simulink model "fir_core"  (Simulink 7.4)
settings: Solver=ode45  StartTime=0.0  StopTime=10.0  RelTol=1e-3
undefined symbols (not defined in the file or in its folder): pfb_coeff_gen_calc
libraries: xbsIndex_r4 x708, casper_library_delays x96
(part 1 of 9)
settings Model: Creator=rprimian  LastModifiedBy=rprimian
settings DebuggingCC: StrictBusMsg=ErrorLevel1

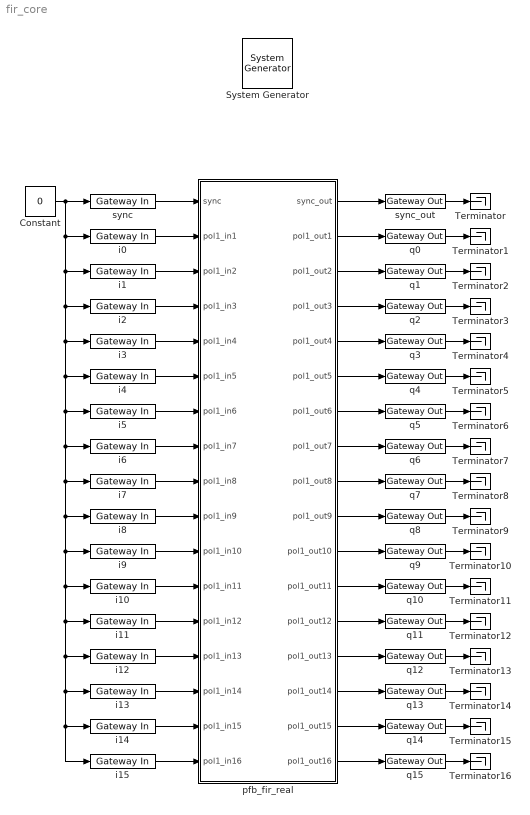
== system fir_core ==
  " System Generator" : xbsIndex_r4/ System Generator  Tag=genX  SystemSampleTime=-1  xilinxfamily=virtex6  part=xc6vsx475t  speed=-1  package=ff1759  synthesis_tool=XST  clock_wrapper=Clock Enables  directory=./fir_core  testbench=off  simulink_period=1  sysclk_period=10  dcm_input_clock_period=100  incr_netlist=off  trim_vbits=Everywhere in SubSystem  dbl_ovrd=According to Block Masks  core_generation=According to Block Masks  run_coregen=off  deprecated_control=off  eval_field=0  block_type=sysgen
      settings: block_version=11.4
  Constant : Constant  Value=0
  Terminator{,1..16} (17 alike) : Terminator
  i{0..15} (16 alike) : xbsIndex_r4/Gateway In  arith_type="Signed  (2's comp)"  n_bits=8  bin_pt=7  quantization="Round  (unbiased: +/- Inf)"  overflow=Saturate  period=1  dbl_ovrd=off  timing_constraint=None  locs_specified=off  LOCs={}  hdl_port=on  block_type=gatewayin
      settings: infoedit="Gateway in block.  Converts inputs of type Simulink integer, double and fixed point to  Xilinx fixed point type.<br><br>Hardware notes:  In hardware these blocks become top level input ports."  block_version=11.4
  pfb_fir_real : Subsystem  AncestorBlock=casper_library_pfbs/pfb_fir_real  mask(pfb_fir_real){PFBSize=15, TotalTaps=4, WindowType=hamming, n_inputs=4, MakeBiplex=off, BitWidthIn=8, BitWidthOut=18, CoeffBitWidth=18, CoeffDistMem=off, add_latency=3, mult_latency=3, bram_latency=3, fan_latency=1, conv_latency=3, quantization=Round  (unbiased: +/- Inf), fwidth=1, mult_spec=2, adder_folding=off, adder_imp=Behavioral, coeffs_share=off}
      mask prompts: PFBSize "Size of PFB: (2^? pnts)"; TotalTaps "Total Number of Taps:"; WindowType "Windowing Function:"; n_inputs "Number of Simultaneous Inputs: (2^?)"; MakeBiplex "Make Biplex?"; BitWidthIn "Input Bitwidth:"; BitWidthOut "Output Bitwidth:"; CoeffBitWidth "Coefficient Bitwidth:"; CoeffDistMem "Use Distributed Memory for Coeffs"; add_latency "Add Latency"; mult_latency "Mult Latency"; bram_latency "BRAM Latency"; fan_latency "Fanout latency"; conv_latency "Convert latency"; quantization "Quantization Behavior"; fwidth "Bin Width Scaling (normal=1)"; mult_spec "Multiplier specification (0=core, 1=embedded, 2=behavioural) (left=1st tap, or just one value)"; adder_folding "Fold adders into DSPs"; adder_imp "Adder implementation"; coeffs_share "Share coefficients between polarisations (use less BRAM)?"
      mask help:
      | Fold adders into DSPs: Causes adders to be absorbed into DSP blocks (supported in Virtex5)
      | Adder implementation: Cores using Fabric or DSP48 or behavioral HDL
      mask init:
      | pfb_fir_real_init(gcb, ...
      |     'PFBSize', PFBSize, ...
      |     'TotalTaps', TotalTaps, ...
      |     'WindowType', WindowType, ...
      |     'n_inputs', n_inputs, ...
      |     'MakeBiplex', MakeBiplex, ...
      |     'BitWidthIn', BitWidthIn, ...
      |     'BitWidthOut', BitWidthOut, ...
      |     'CoeffBitWidth', CoeffBitWidth, ...
      |     'CoeffDistMem', CoeffDistMem, ...
      |     'add_latency', add_latency, ...
      |     'mult_latency', mult_latency, ...
      |     'bram_latency', bram_latency, ...
      |     'fan_latency', fan_latency, ...
      |     'conv_latency', conv_latency, ...
      |     'quantization', quantization, ...
      |     'fwidth', fwidth, ...
      |     'mult_spec', mult_spec, ...
      |     'adder_folding', adder_folding, ...
      |     'adder_imp', adder_imp, ...
      |     'coeffs_share', coeffs_share);
      settings: AttributesFormatString=taps=4, add_latency=3
      mask Help: eval('xlWeb(''http://casper.berkeley.edu/wiki/Pfb_fir_real'')')
      mask StyleString: edit,edit,popup(bartlett|barthannwin|blackman|blackmanharris|bohamwin|chebwin|flattopwin|gausswin|hamming|hann|kaiser|nuttallwin|parzenwin|rectwin|tukeywin|triang|userwindow),edit,checkbox,edit,edit,edit,checkbox,edit,edit,edit,edit,edit,popup(Truncate|Round  (unbiased: +/- Inf)|Round  (unbiased: Even Values)),edit,edit,checkbox,popup(Behavioral|Fabric|DSP48),checkbox
      mask CallbackString:
      | |%num_taps = eval(get_param(gcb, 'TotalTaps'));
      | %old_vec = eval(get_param(gcb, 'mult_spec'));=-0l
      | 
      | %vec = 2.*ones(1,num_taps);
      | %old_size = length(old_vec);
      | 
      | %if(old_size <= num_taps),
      | %    new_size = old_size;
      | %else,
      | %    new_size = num_taps;
      | %end
      | 
      | %for n = 1:new_size, vec(n) = old_vec(n); end
      | %set_param(gcb, 'mult_spec', mat2str(vec));||||||||||||||||||
  q{0..15} (16 alike) : xbsIndex_r4/Gateway Out  hdl_port=on  timing_constraint=None  locs_specified=off  LOCs={}  block_type=gatewayout
      settings: infoedit="Gateway out block.  Converts Xilinx fixed point inputs into ouputs of type Simulink integer, double, or fixed point.<br><br>Hardware notes:  In hardware these blocks become top level output ports or are discarded, depending on how they are configured."  block_version=11.4
  sync : xbsIndex_r4/Gateway In  arith_type=Boolean  n_bits=1  bin_pt=0  quantization="Round  (unbiased: +/- Inf)"  overflow=Saturate  period=1  dbl_ovrd=off  timing_constraint=None  locs_specified=off  LOCs={}  hdl_port=on  block_type=gatewayin
      settings: infoedit="Gateway in block.  Converts inputs of type Simulink integer, double and fixed point to  Xilinx fixed point type.<br><br>Hardware notes:  In hardware these blocks become top level input ports."  block_version=11.4
  sync_out : xbsIndex_r4/Gateway Out  hdl_port=on  timing_constraint=None  locs_specified=off  LOCs={}  block_type=gatewayout
      settings: infoedit="Gateway out block.  Converts Xilinx fixed point inputs into ouputs of type Simulink integer, double, or fixed point.<br><br>Hardware notes:  In hardware these blocks become top level output ports or are discarded, depending on how they are configured."  block_version=11.4
  wires:
  sync/1 -> pfb_fir_real/1(sync)
  i0/1 -> pfb_fir_real/2(pol1_in1)
  i1/1 -> pfb_fir_real/3(pol1_in2)
  i2/1 -> pfb_fir_real/4(pol1_in3)
  i3/1 -> pfb_fir_real/5(pol1_in4)
  i4/1 -> pfb_fir_real/6(pol1_in5)
  i5/1 -> pfb_fir_real/7(pol1_in6)
  i6/1 -> pfb_fir_real/8(pol1_in7)
  i7/1 -> pfb_fir_real/9(pol1_in8)
  i8/1 -> pfb_fir_real/10(pol1_in9)
  i9/1 -> pfb_fir_real/11(pol1_in10)
  i10/1 -> pfb_fir_real/12(pol1_in11)
  i11/1 -> pfb_fir_real/13(pol1_in12)
  i12/1 -> pfb_fir_real/14(pol1_in13)
  i13/1 -> pfb_fir_real/15(pol1_in14)
  i14/1 -> pfb_fir_real/16(pol1_in15)
  i15/1 -> pfb_fir_real/17(pol1_in16)
  Constant/1 -> sync/1, i0/1, i1/1, i2/1, i3/1, i4/1, i5/1, i6/1, i7/1, i8/1, i9/1, i10/1, i11/1, i12/1, i13/1, i14/1, i15/1
  pfb_fir_real/1(sync_out) -> sync_out/1
  sync_out/1 -> Terminator/1
  q0/1 -> Terminator1/1
  q1/1 -> Terminator2/1
  q2/1 -> Terminator3/1
  q3/1 -> Terminator4/1
  q4/1 -> Terminator5/1
  q5/1 -> Terminator6/1
  q6/1 -> Terminator7/1
  q7/1 -> Terminator8/1
  q8/1 -> Terminator9/1
  q9/1 -> Terminator10/1
  q10/1 -> Terminator11/1
  q11/1 -> Terminator12/1
  q12/1 -> Terminator13/1
  q13/1 -> Terminator14/1
  q14/1 -> Terminator15/1
  q15/1 -> Terminator16/1
  pfb_fir_real/2(pol1_out1) -> q0/1
  pfb_fir_real/3(pol1_out2) -> q1/1
  pfb_fir_real/4(pol1_out3) -> q2/1
  pfb_fir_real/5(pol1_out4) -> q3/1
  pfb_fir_real/6(pol1_out5) -> q4/1
  pfb_fir_real/7(pol1_out6) -> q5/1
  pfb_fir_real/8(pol1_out7) -> q6/1
  pfb_fir_real/9(pol1_out8) -> q7/1
  pfb_fir_real/10(pol1_out9) -> q8/1
  pfb_fir_real/11(pol1_out10) -> q9/1
  pfb_fir_real/12(pol1_out11) -> q10/1
  pfb_fir_real/13(pol1_out12) -> q11/1
  pfb_fir_real/14(pol1_out13) -> q12/1
  pfb_fir_real/15(pol1_out14) -> q13/1
  pfb_fir_real/16(pol1_out15) -> q14/1
  pfb_fir_real/17(pol1_out16) -> q15/1
